simulink subsystem "WindGenerator"  (R2023b)
settings: Solver=VariableStepAuto  StartTime=0.0  StopTime=10.0  RelTol=1e-3
values from neighbouring files (symbols this model uses):
  laz = 1.612    [Diplomm.m]
  lel = 1.586    [Diplomm.m]
settings Model: Creator=mrrom  LastModifiedBy=mrrom

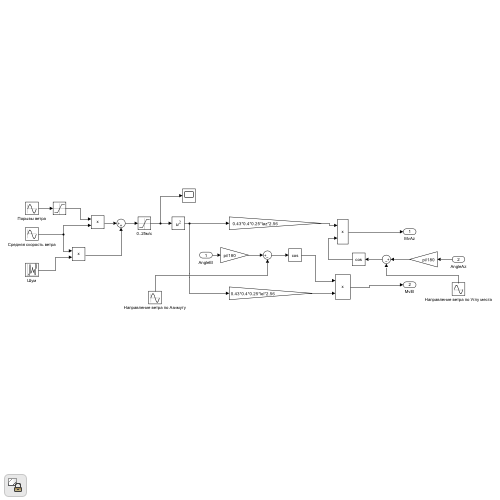
[thumbnail: Simulink's stored preview of the top-level diagram]
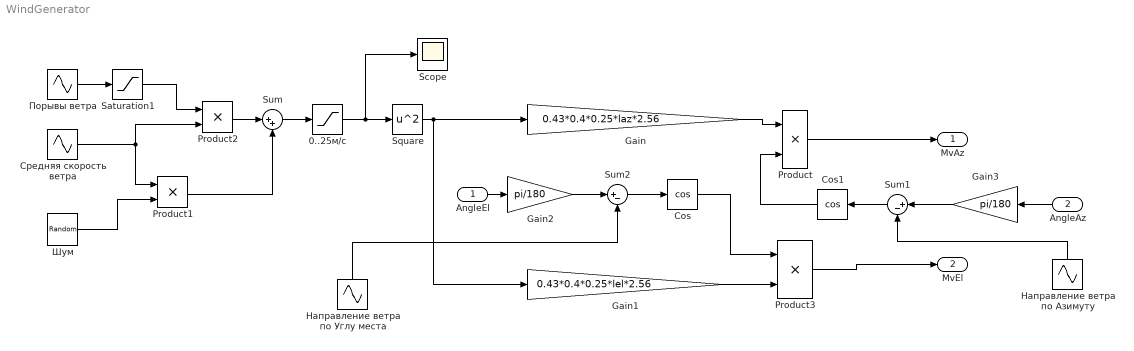
== system WindGenerator ==
  AngleEl : Inport
  AngleAz : Inport  Port=2
  0..25м/c : Saturate  UpperLimit=25  LowerLimit=0
  Cos : Trigonometry  Operator=cos
  Cos1 : Trigonometry  Operator=cos
  Gain : Gain  Gain=0.43*0.4*0.25*laz*2.56
  Gain1 : Gain  Gain=0.43*0.4*0.25*lel*2.56
  Gain2 : Gain  Gain=pi/180
  Gain3 : Gain  Gain=pi/180
  Product{,1..3} (4 alike) : Product
  Saturation1 : Saturate  LowerLimit=0
  Scope : Scope
  Square : Math  Operator=square
  Sum : Sum  Inputs=|++
  Sum1 : Sum  Inputs=|+-
  Sum2 : Sum  Inputs=|+-
  "Направление ветра по Азимуту " : Sin  Amplitude=pi  Frequency=1.16e-3  Phase=pi/4  SampleTime=0
  Направление ветра по Углу места : Sin  Amplitude=pi/2  Frequency=1.16e-3  SampleTime=0
  Порывы ветра : Sin  Amplitude=0.5  Frequency=1.4  Phase=pi/2  SampleTime=0
  Средняя скорость ветра : Sin  Amplitude=0.5  Bias=2  Frequency=0.1  SampleTime=0
  Шум : UniformRandomNumber  Maximum=10  SampleTime=10.8
  MvAz : Outport
  MvEl : Outport  Port=2
  wires:
  Product/1 -> MvAz/1
  AngleEl/1 -> Gain2/1
  0..25м/c/1 -> Square/1, Scope/1
  Средняя скорость ветра/1 -> Product1/1, Product2/2
  Шум/1 -> Product1/2
  Gain/1 -> Product/1
  Square/1 -> Gain1/1, Gain/1
  Cos/1 -> Product3/1
  Product1/1 -> Sum/2
  Порывы ветра/1 -> Saturation1/1
  Product2/1 -> Sum/1
  Saturation1/1 -> Product2/1
  Sum/1 -> 0..25м/c/1
  Product3/1 -> MvEl/1
  AngleAz/1 -> Gain3/1
  Cos1/1 -> Product/2
  Gain3/1 -> Sum1/1
  Sum1/1 -> Cos1/1
  Gain2/1 -> Sum2/1
  Sum2/1 -> Cos/1
  Направление ветра по Углу места/1 -> Sum2/2
  Gain1/1 -> Product3/2
  "Направление ветра по Азимуту "/1 -> Sum1/2
